simulink library "INT_PSPCtl_Co"  (R2016b)
settings: Solver=VariableStepAuto  StartTime=0.0  StopTime=10.0  RelTol=1e-3
settings Model: Creator=liutao  LastModifiedBy=liutao

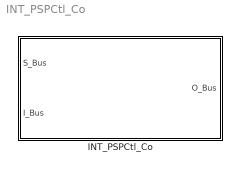
== system INT_PSPCtl_Co ==
  INT_PSPCtl_Co : Subsystem

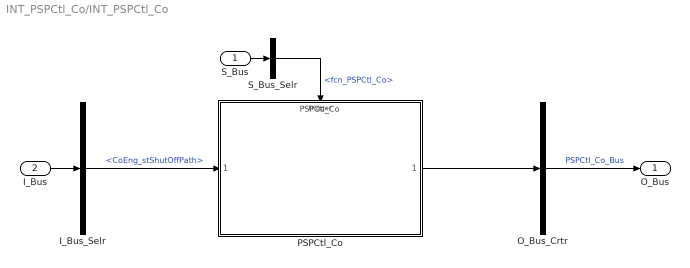
== system INT_PSPCtl_Co/INT_PSPCtl_Co ==
  S_Bus : Inport
  I_Bus : Inport  Port=2
  I_Bus_Selr : BusSelector  OutputSignals=CoEng_stShutOffPath
  O_Bus_Crtr : BusCreator  Inputs=1
  PSPCtl_Co : ModelReference  ModelNameDialog=PSPCtl_Co  SimulationMode=Normal  ModelReferenceVersion=1.7  TriggerPortName=function  TriggerPortTriggerType=function-call  TriggerPortStatesWhenEnabling=held
  S_Bus_Selr : BusSelector  OutputSignals=fcn_PSPCtl_Co
  O_Bus : Outport
  wires:
  S_Bus_Selr/1 -> PSPCtl_Co/Trigger  "<fcn_PSPCtl_Co>"
  S_Bus/1 -> S_Bus_Selr/1
  I_Bus/1 -> I_Bus_Selr/1
  I_Bus_Selr/1 -> PSPCtl_Co/1  "<CoEng_stShutOffPath>"
  O_Bus_Crtr/1 -> O_Bus/1  "PSPCtl_Co_Bus"
  PSPCtl_Co/1 -> O_Bus_Crtr/1
